simulink model "HMI_p8"  (R2017a)
settings: Solver=VariableStepAuto  StartTime=0.0  StopTime=10.0  RelTol=1e-3
libraries: powerlib_meascontrol x2, vrlib x1
settings Model: Creator=GABI  LastModifiedBy=GABI

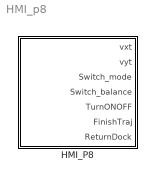
== system HMI_p8 ==
  HMI_P8 : Subsystem

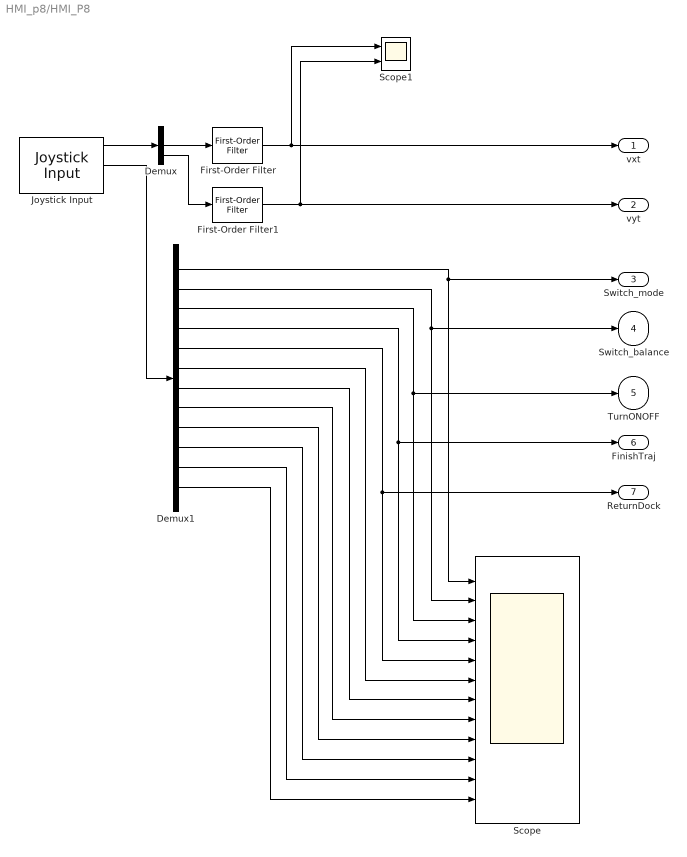
== system HMI_p8/HMI_P8 ==
  Demux : Demux  Outputs=3
  Demux1 : Demux  Outputs=12
  First-Order Filter : powerlib_meascontrol/Filters/First-Order Filter  FilterType=Lowpass  Tc=10e-3  Ts=0  Initialize=off  Vac_Init=[0, 0, 60]  Vdc_Init=0  PlotResponse=off  FreqRange="[0,  200,  1]"
      settings: SourceProductName=Simscape Power Systems
  First-Order Filter1 : powerlib_meascontrol/Filters/First-Order Filter  FilterType=Lowpass  Tc=10e-3  Ts=0  Initialize=off  Vac_Init=[0, 0, 60]  Vdc_Init=0  PlotResponse=off  FreqRange="[0,  200,  1]"
      settings: SourceProductName=Simscape Power Systems
  Joystick Input : vrlib/Joystick Input  joyid=1  adjustports=on  forcefeed=off
      settings: SourceProductBaseCode=VR
  Scope : Scope  NumInputPorts=12
  Scope1 : Scope  NumInputPorts=2
  vxt : Outport
  vyt : Outport  Port=2
  Switch_mode : Outport  Port=3
  Switch_balance : Outport  Port=4
  TurnONOFF : Outport  Port=5
  FinishTraj : Outport  Port=6
  ReturnDock : Outport  Port=7
  wires:
  First-Order Filter1/1 -> Scope1/2, vyt/1
  First-Order Filter/1 -> Scope1/1, vxt/1
  Joystick Input/2 -> Demux1/1
  Demux/2 -> First-Order Filter/1
  Demux/3 -> First-Order Filter1/1
  Demux1/1 -> Switch_mode/1, Scope/1
  Demux1/2 -> Switch_balance/1, Scope/2
  Demux1/3 -> TurnONOFF/1, Scope/3
  Demux1/4 -> FinishTraj/1, Scope/4
  Demux1/5 -> ReturnDock/1, Scope/5
  Demux1/6 -> Scope/6
  Demux1/7 -> Scope/7
  Demux1/8 -> Scope/8
  Demux1/9 -> Scope/9
  Demux1/10 -> Scope/10
  Demux1/11 -> Scope/11
  Demux1/12 -> Scope/12
  Joystick Input/1 -> Demux/1
